simulink model "double_shared_torque"  (R2019b)
settings: Solver=FixedStepAuto  StartTime=0.0  StopTime=10.0  FixedStep=.01  RelTol=1e-3
values from neighbouring files (symbols this model uses):
  Ked = [ 500, 0; 0, 500]    [double_pend_setup.m]    (also in double_pend_varible_setup.m = [ 50, 0; 0, 50]; double_with_kalman.m = [ 50, 0; 0, 50]; testing_Exo_setup.m = [ 50, 0; 0, 50])
  Kem = [500, 0; 0, 500]    [double_pend_setup.m]    (also in double_pend_varible_setup.m = [ 50, 0; 0, 50]; double_with_kalman.m = [ 50, 0; 0, 50]; testing_Exo_setup.m = [ 50, 0; 0, 50])
  l = [ 1.0, 1.5]    [double_pend_setup.m]    (also in double_pend_varible_setup.m; double_with_kalman.m; myStateTransitionFcn.m = [0.324, 0.3900]; testing_Exo_setup.m = [0.324, 0.3900])
  me = [ 5, 5] + mh    [double_pend_setup.m]    (also in double_pend_varible_setup.m = [ 1, 1] + mh; double_with_kalman.m; testing_Exo_setup.m = [ 2.11, 1.28]  + mh)
  mh = [2, 1]    [double_pend_setup.m]    (also in double_pend_varible_setup.m; double_with_kalman.m; testing_Exo_setup.m = [11.824, 3.848])
undefined symbols (not defined in the file or in its folder): l1, l2, me2
libraries: robotcorelib x1
settings Model: Creator=nathanielgoldfarb  LastModifiedBy=nathanielgoldfarb

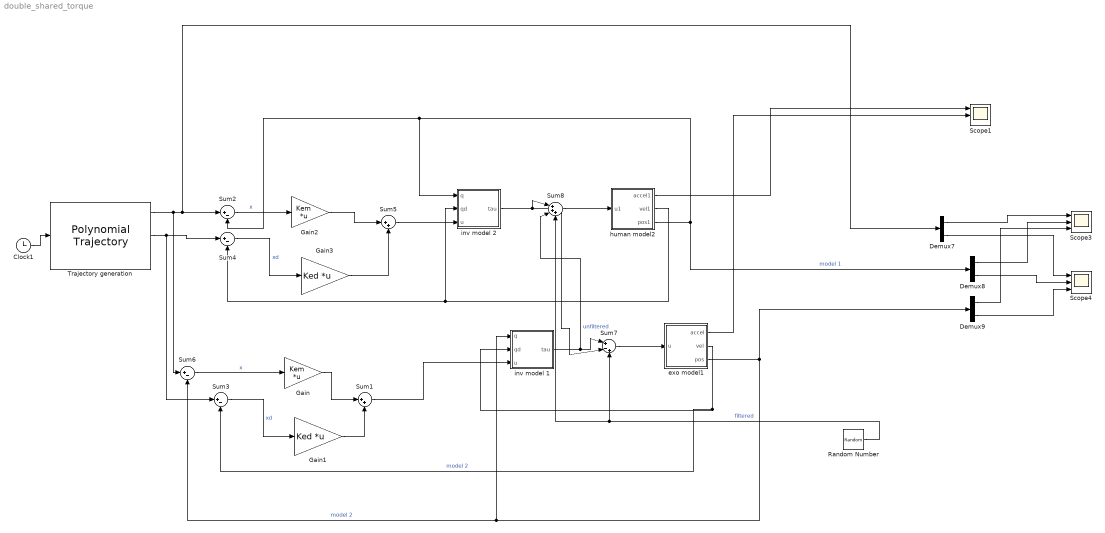
== system double_shared_torque ==
  Clock1 : Clock
  Demux7 : Demux  Outputs=2
  Demux8 : Demux  Outputs=2
  Demux9 : Demux  Outputs=2
  Gain : Gain  Gain=Kem  Multiplication=Matrix(K*u)
  Gain1 : Gain  Gain=Ked  Multiplication=Matrix(K*u)
  Gain2 : Gain  Gain=Kem  Multiplication=Matrix(K*u)
  Gain3 : Gain  Gain=Ked  Multiplication=Matrix(K*u)
  Random Number : RandomNumber  Variance=20  SampleTime=0.1
  Scope1 : Scope  NumInputPorts=3
  Scope3 : Scope  NumInputPorts=3
  Scope4 : Scope  NumInputPorts=3
  Sum1 : Sum  Inputs=|++
  Sum{2..4,6} (4 alike) : Sum  Inputs=|+-
  Sum5 : Sum  Inputs=|++
  Sum7 : Sum  Inputs=|+-+
  Sum8 : Sum  Inputs=|+++
  Trajectory generation : robotcorelib/Polynomial Trajectory  WaypointSource=Internal  Waypoints="[ 0 , -pi 0;  0 -0.5*pi 0 ]"  TimePoints=[ 0, 5, 10]  TimeInterval=[ 1, 4 ]  Method=Cubic Polynomial  ParameterSource=Internal  VelocityBoundaryCondition=zeros( 2, 3 )  AccelerationBoundaryCondition=zeros( 2, 5 )  SimulateUsing=Interpreted execution
      settings: SourceProductName=Robotics System Toolbox  SourceProductBaseCode=RO
  exo model1 : Subsystem
  human model2 : Subsystem
  inv model 1 : Subsystem
  inv model 2 : Subsystem
  wires:
  Demux7/2 -> Scope4/1
  Sum3/1 -> Gain1/1  "xd"
  Sum6/1 -> Gain/1  "x"
  Demux9/2 -> Scope4/3
  inv model 1/1("tau ") -> Sum8/2, Sum7/1  "unfiltered"
  Sum1/1 -> inv model 1/3("u ")
  Demux8/1 -> Scope3/2
  exo model1/2(vel) -> Sum3/2, inv model 1/2(qd)  "model 2"
  Demux8/2 -> Scope4/2
  human model2/3(pos1) -> inv model 2/1(q), Sum2/2, Demux8/1  "model 1"
  Sum7/1 -> exo model1/1(u)
  Gain1/1 -> Sum1/2
  Clock1/1 -> Trajectory generation/1
  Gain/1 -> Sum1/1
  Demux9/1 -> Scope3/3
  Demux7/1 -> Scope3/1
  exo model1/3(pos) -> Sum6/2, inv model 1/1(q), Demux9/1  "model 2"
  Sum2/1 -> Gain2/1  "x"
  Sum4/1 -> Gain3/1  "xd"
  Trajectory generation/1 -> Sum6/1, Demux7/1, Sum2/1
  Trajectory generation/2 -> Sum3/1, Sum4/1
  Gain2/1 -> Sum5/1
  Gain3/1 -> Sum5/2
  Sum5/1 -> inv model 2/3("u ")
  human model2/2(vel1) -> inv model 2/2(qd), Sum4/2
  inv model 2/1("tau ") -> Sum7/2, Sum8/1
  Random Number/1 -> Sum7/3, Sum8/3  "filtered"
  Sum8/1 -> human model2/1(u1)
  human model2/1(accel1) -> Scope1/1
  exo model1/1(accel) -> Scope1/2

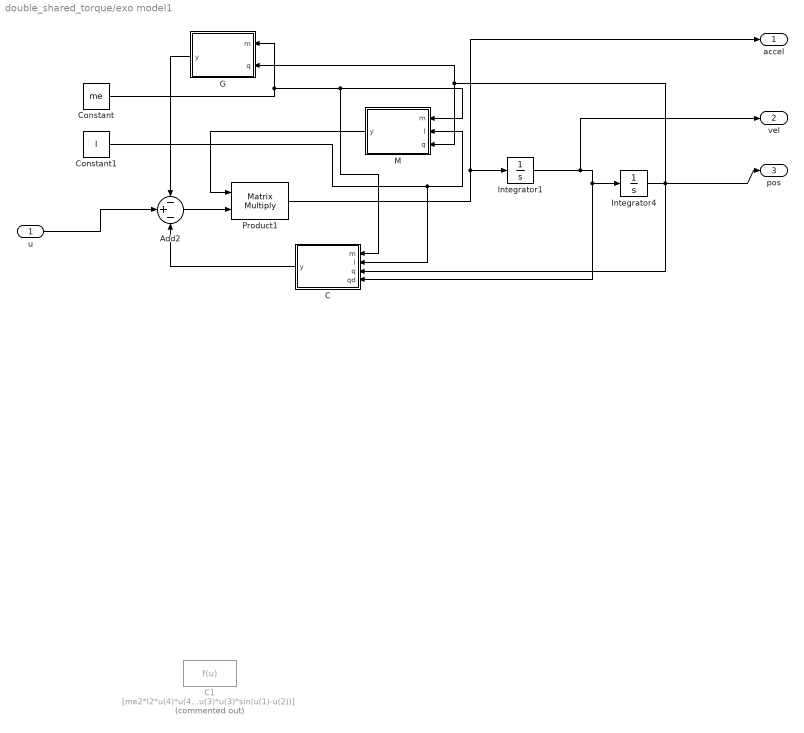
== system double_shared_torque/exo model1 ==
  u : Inport
  Add2 : Sum  Inputs=-+-
  C : MATLAB Function  TreatAsAtomicUnit=on
  C1 : Fcn  Commented=on  Expr=[me2*l2*u(4)*u(4)*sin(u(1)-u(2)); -me2*l1*u(3)*u(3)*sin(u(1)-u(2))]
  Constant : Constant  Value=me
  Constant1 : Constant  Value=l
  G : MATLAB Function  TreatAsAtomicUnit=on
  Integrator1 : Integrator  InitialCondition=[0;0]
  Integrator4 : Integrator  InitialCondition=[0.1;0.1]
  M : MATLAB Function  TreatAsAtomicUnit=on
  Product1 : Product  Multiplication=Matrix(*)
  accel : Outport
  vel : Outport  Port=2
  pos : Outport  Port=3
  wires:
  Constant/1 -> G/1(m), C/1(m), M/1(m)
  M/1(y) -> Product1/1
  Add2/1 -> Product1/2
  C/1(y) -> Add2/3
  G/1(y) -> Add2/1
  u/1 -> Add2/2
  Product1/1 -> accel/1, Integrator1/1
  Constant1/1 -> C/2(l), M/2(l)
  Integrator1/1 -> vel/1, C/4(qd), Integrator4/1
  Integrator4/1 -> C/3(q), pos/1, M/3(q), G/2(q)

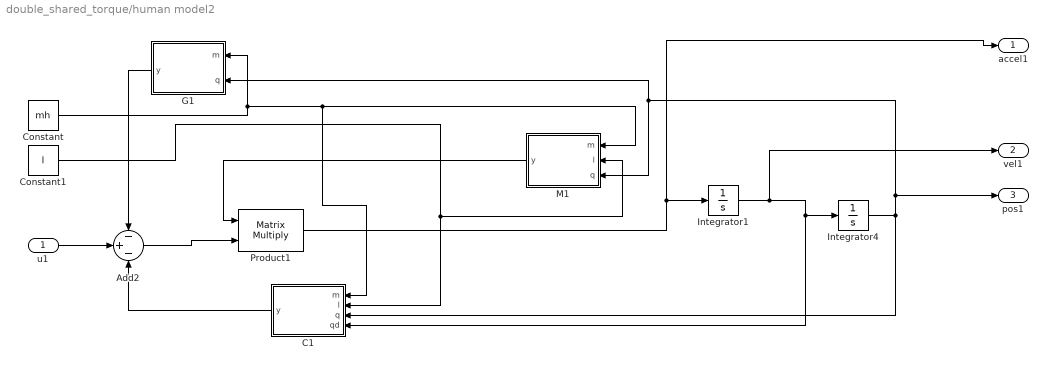
== system double_shared_torque/human model2 ==
  u1 : Inport
  Add2 : Sum  Inputs=-+-
  C1 : MATLAB Function  TreatAsAtomicUnit=on
  Constant : Constant  Value=mh
  Constant1 : Constant  Value=l
  G1 : MATLAB Function  TreatAsAtomicUnit=on
  Integrator1 : Integrator  InitialCondition=[0;0]
  Integrator4 : Integrator  InitialCondition=[0.1;0.1]
  M1 : MATLAB Function  TreatAsAtomicUnit=on
  Product1 : Product  Multiplication=Matrix(*)
  accel1 : Outport
  vel1 : Outport  Port=2
  pos1 : Outport  Port=3
  wires:
  C1/1(y) -> Add2/3
  M1/1(y) -> Product1/1
  G1/1(y) -> Add2/1
  Integrator4/1 -> C1/3(q), pos1/1, M1/3(q), G1/2(q)
  u1/1 -> Add2/2
  Product1/1 -> accel1/1, Integrator1/1
  Integrator1/1 -> vel1/1, C1/4(qd), Integrator4/1
  Add2/1 -> Product1/2
  Constant/1 -> G1/1(m), C1/1(m), M1/1(m)
  Constant1/1 -> C1/2(l), M1/2(l)

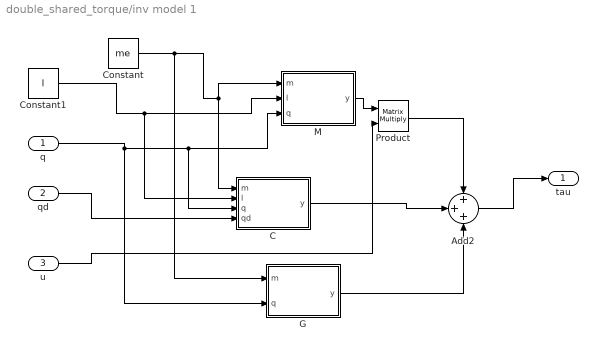
== system double_shared_torque/inv model 1 ==
  q : Inport
  qd : Inport  Port=2
  "u " : Inport  Port=3
  Add2 : Sum  Inputs=+++
  C : MATLAB Function  TreatAsAtomicUnit=on
  Constant : Constant  Value=me
  Constant1 : Constant  Value=l
  G : MATLAB Function  TreatAsAtomicUnit=on
  M : MATLAB Function  TreatAsAtomicUnit=on
  Product : Product  Multiplication=Matrix(*)
  "tau " : Outport
  wires:
  G/1(y) -> Add2/3
  C/1(y) -> Add2/2
  q/1 -> G/2(q), M/3(q), C/3(q)
  qd/1 -> C/4(qd)
  M/1(y) -> Product/1
  Product/1 -> Add2/1
  Constant/1 -> G/1(m), M/1(m), C/1(m)
  Constant1/1 -> M/2(l), C/2(l)
  "u "/1 -> Product/2
  Add2/1 -> "tau "/1

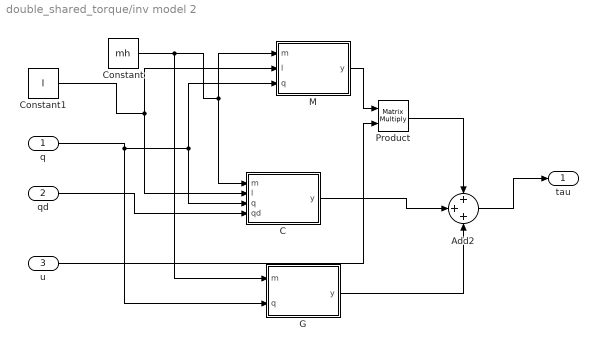
== system double_shared_torque/inv model 2 ==
  q : Inport
  qd : Inport  Port=2
  "u " : Inport  Port=3
  Add2 : Sum  Inputs=+++
  C : MATLAB Function  TreatAsAtomicUnit=on
  Constant : Constant  Value=mh
  Constant1 : Constant  Value=l
  G : MATLAB Function  TreatAsAtomicUnit=on
  M : MATLAB Function  TreatAsAtomicUnit=on
  Product : Product  Multiplication=Matrix(*)
  "tau " : Outport
  wires:
  Constant1/1 -> C/2(l), M/2(l)
  Constant/1 -> G/1(m), C/1(m), M/1(m)
  "u "/1 -> Product/2
  Product/1 -> Add2/1
  M/1(y) -> Product/1
  qd/1 -> C/4(qd)
  q/1 -> G/2(q), C/3(q), M/3(q)
  Add2/1 -> "tau "/1
  C/1(y) -> Add2/2
  G/1(y) -> Add2/3

== matlab function double_shared_torque/inv model 2/C ==
  data: m input; l input; q input; y output; qd input
function y = fcn(m, l, q, qd)



y = C(m, l, q, qd); % [m(2)*l(2)*qd(2)*qd(2)*sin(q(1)-q(2)); -m(2)*l(1)*qd(1)*qd(1)*sin(q(1)-q(2))];

== matlab function double_shared_torque/inv model 2/G ==
  data: m input; q input; y output
function y = fcn(m, q)
 y =  G(m,q);
end

== matlab function double_shared_torque/inv model 2/M ==
  data: m input; l input; q input; y output
function y = fcn(m, l, q)

y = M(m,l,q); % pinv([ (m(1)+m(2)) *l(1), m(2)*l(2)*cos(q(1)-q(2)); m(2)* l(1)*cos(q(1)-q(2)), m(2)*l(2)] );

end

== matlab function double_shared_torque/inv model 1/C ==
  data: m input; l input; q input; y output; qd input
function y = fcn(m, l, q, qd)



y = C(m, l, q, qd); % [m(2)*l(2)*qd(2)*qd(2)*sin(q(1)-q(2)); -m(2)*l(1)*qd(1)*qd(1)*sin(q(1)-q(2))];

== matlab function double_shared_torque/inv model 1/G ==
  data: m input; q input; y output
function y = fcn(m, q)
 y =  G(m,q);
end

== matlab function double_shared_torque/inv model 1/M ==
  data: m input; l input; q input; y output
function y = fcn(m, l, q)

y = M(m,l,q); % pinv([ (m(1)+m(2)) *l(1), m(2)*l(2)*cos(q(1)-q(2)); m(2)* l(1)*cos(q(1)-q(2)), m(2)*l(2)] );

end

== matlab function double_shared_torque/exo model1/C ==
  data: m input; l input; q input; y output; qd input
function y = fcn(m, l, q, qd)



y = C(m, l, q, qd); % [m(2)*l(2)*qd(2)*qd(2)*sin(q(1)-q(2)); -m(2)*l(1)*qd(1)*qd(1)*sin(q(1)-q(2))];

== matlab function double_shared_torque/exo model1/G ==
  data: m input; q input; y output
function y = fcn(m, q)
 y = [50;50] + G(m,q);
end

== matlab function double_shared_torque/exo model1/M ==
  data: m input; l input; q input; y output
function y = fcn(m, l, q)

y = pinv(M(m,l,q)); % pinv([ (m(1)+m(2)) *l(1), m(2)*l(2)*cos(q(1)-q(2)); m(2)* l(1)*cos(q(1)-q(2)), m(2)*l(2)] );

end

== matlab function double_shared_torque/human model2/C1 ==
  data: m input; l input; q input; y output; qd input
function y = fcn(m, l, q, qd)



y = C(m, l, q, qd); % [m(2)*l(2)*qd(2)*qd(2)*sin(q(1)-q(2)); -m(2)*l(1)*qd(1)*qd(1)*sin(q(1)-q(2))];

== matlab function double_shared_torque/human model2/G1 ==
  data: m input; q input; y output
function y = fcn(m, q)
 y =  G(m,q);
end

== matlab function double_shared_torque/human model2/M1 ==
  data: m input; l input; q input; y output
function y = fcn(m, l, q)

y = pinv(M(m,l,q)); % pinv([ (m(1)+m(2)) *l(1), m(2)*l(2)*cos(q(1)-q(2)); m(2)* l(1)*cos(q(1)-q(2)), m(2)*l(2)] );

end
